simulink model "gm_Model"  (R2025a)
settings: Solver=FixedStepDiscrete  StartTime=0.0  StopTime=80000/fs_in  RelTol=1e-3
undefined symbols (not defined in the file or in its folder): a, b, b_fixp, beta_retanh, c, cos_omega, cos_omega_fixp, diag_count, exp_omega, exp_omega_fixp, fixp_chebacc_frac, fixp_chebacc_ws, fixp_dsp_ws, fixp_eig_frac, fixp_eig_ws, fs_in, group_size, hann_table_fixp, image_seed, image_seed_fixp, J_ROM, k, K_ROM, lap_diags, lap_main, lap_main_fi, lap_offsets, lap_offsets_fi, lap_rest, lap_rest_fi, laplacian_diags_main, laplacian_diags_offsets, laplacian_diags_rest, lut_norm_x, lut_norm_y, magnitude, n_ch, n_layer, n_px, n_px_fi, nf, norm_gain_floor, power_iters, power_norm_scaling_factor_fixp, tau, tau_fixp, theta, theta_fixp
libraries: simulink x59, hdlsllib x36, hdlstreaminglib x4, hdlmdlgenlib x1, matrix_library x1, dspvision x1
(part 8 of 8)

== system gm_Model/DUT_Test/Goertzel/EnabledGoertzel/streaming_partition_streamed2/tappedDelay ==
  in0 : Inport  OutDataTypeStr=fixdt(1, 18, 13)  SampleTime=3.125e-07
      settings: SignalType=complex
  globalSchedule : EnablePort  OutDataTypeStr=boolean
  StateControl : StateControl  StateControl=Synchronous
  tapped_delay : simulink/Discrete/Tapped Delay  vinit=0  samptime=-1  NumDelays=double(47)  DelayOrder=Oldest  includeCurrent=off
  out0 : Outport  OutDataTypeStr=fixdt(1, 18, 13)  PortDimensions=[47]  SampleTime=3.125e-07  InitialOutput=0
      settings: SignalType=complex
  wires:
  in0/1 -> tapped_delay/1
  tapped_delay/1 -> out0/1

== system gm_Model/DUT_Test/Goertzel/EnabledGoertzel/streaming_partition_streamed2/tappedDelay1 ==
  in0 : Inport  OutDataTypeStr=fixdt(1, 18, 13)  SampleTime=3.125e-07
      settings: SignalType=complex
  globalSchedule : EnablePort  OutDataTypeStr=boolean
  StateControl : StateControl  StateControl=Synchronous
  tapped_delay : simulink/Discrete/Tapped Delay  vinit=0  samptime=-1  NumDelays=double(47)  DelayOrder=Oldest  includeCurrent=off
  out0 : Outport  OutDataTypeStr=fixdt(1, 18, 13)  PortDimensions=[47]  SampleTime=3.125e-07  InitialOutput=0
      settings: SignalType=complex
  wires:
  in0/1 -> tapped_delay/1
  tapped_delay/1 -> out0/1

== system gm_Model/DUT_ref/CrossCor/Grouping/DataValidDownsampler/RisingEdgeDetector ==
  In1 : Inport
  AND : Logic  IconShape=distinctive  AllPortsSameDT=off  OutDataTypeStr=boolean
  Delay1 : Delay  DelayLength=1
  NOT : Logic  Operator=NOT  IconShape=distinctive  AllPortsSameDT=off  OutDataTypeStr=boolean
  Out1 : Outport
  wires:
  Delay1/1 -> NOT/1
  AND/1 -> Out1/1
  NOT/1 -> AND/1
  In1/1 -> AND/2, Delay1/1

== system gm_Model/DUT_ref/Deblurring/Chebyshev/LaplacianMultiply/For Each Subsystem ==
  note: This is too slow in simulation... Might be more suitable for HDL coder though (not checked)
  note: Main Diagonal
  note: Lower triangle
  note: Upper triangle
  ToIterate : Inport  Partition=on  PartitionDimension=1  PartitionWidth=1  PartitionOffset=0
  Image : Inport  Port=2
  Diag : Inport  Port=3
  Offset : Inport  Port=4
  Dot Product : DotProduct  OutDataTypeStr=Inherit: Inherit via internal rule
  Dot Product1 : DotProduct  OutDataTypeStr=Inherit: Inherit via internal rule
  For Each : ForEach  DisableCoverage=on  ShowIterationIndex=on
  IndexedSelector : Subsystem  Commented=on  TreatAsAtomicUnit=on
  MATLAB Function : MATLAB Function  TreatAsAtomicUnit=on
  Product : Product
  Selector{,1,3,5} (4 alike) : Selector  IndexMode=Zero-based  InputPortWidth=n_px  IndexOptions=Index vector (port)  Indices=[1 3]  OutputSizes=1
  Selector4 : Selector  NumberOfDimensions=2  IndexMode=Zero-based  InputPortWidth=n_px  IndexOptions=Select all,Index vector (port)  Indices=[1 3],1  OutputSizes=1,1
  SplitDiagonals : Subsystem
  Sum1 : Sum  Inputs=++|
  Sum2 : Sum  Inputs=-+|  OutDataTypeStr=uint16  SaturateOnIntegerOverflow=on
  Sum3 : Sum  Inputs=+++
  Terminator : Terminator
  Wrap To Zero : hdlsllib/Discontinuities/Wrap To Zero  Threshold=n_px-1
  Image_out : Outport  ConcatenationDimension=1
  wires:
  MATLAB Function/1(out) -> Dot Product/2
  Sum3/1 -> Image_out/1
  Dot Product/1 -> Sum3/3
  Product/1 -> Sum3/1
  Sum2/1 -> Selector5/2
  For Each/1 -> Sum1/2, Selector4/2, Selector1/2, Selector/2, Sum2/2
  Selector5/1 -> Dot Product1/1
  Dot Product1/1 -> Sum3/2
  SplitDiagonals/2(Rest) -> IndexedSelector/1(diags), MATLAB Function/1(data_matrix), Selector4/1
  Offset/1 -> Sum2/1, Sum1/1
  Selector4/1 -> Dot Product1/2
  Selector3/1 -> Dot Product/1
  Wrap To Zero/1 -> IndexedSelector/2(indices), MATLAB Function/2(col_indices), Selector3/2
  Sum1/1 -> Wrap To Zero/1
  ToIterate/1 -> Terminator/1
  SplitDiagonals/1(Main) -> Selector/1
  Selector/1 -> Product/2
  Selector1/1 -> Product/1
  Diag/1 -> SplitDiagonals/1(Diag)
  Image/1 -> Selector5/1, Selector3/1, Selector1/1

== system gm_Model/DUT_ref/Goertzel/EnabledGoertzel/Goertzel filter/For All Bins Filter ==
  In1 : Inport
  Delay : Delay  DelayLength=1
  Delay1 : Delay  DelayLength=1
  For Each : ForEach  DisableCoverage=on  IterateSubsysMaskParameter=on,on  SubsysMaskParameterIterationDimension=2,2
  Multiply1 : Gain  Gain=cos_omega
  Multiply2 : Gain  Gain=exp_omega
  Sum : Sum  Inputs=++-
  Sum1 : Sum  Inputs=|-+
  Out1 : Outport  ConcatenationDimension=1
  wires:
  Delay/1 -> Sum1/2, Sum/3
  Delay1/1 -> Multiply1/1, Multiply2/1, Delay/1
  Multiply2/1 -> Sum1/1
  Multiply1/1 -> Sum/1
  Sum1/1 -> Out1/1
  Sum/1 -> Delay1/1
  In1/1 -> Sum/2

== system gm_Model/DUT_ref/Deblurring/Chebyshev/LaplacianMultiply/For Each Subsystem/IndexedSelector ==
  diags : Inport  Partition=on  PartitionDimension=1  PartitionWidth=1  PartitionOffset=0
  indices : Inport  Port=2  Partition=on  PartitionDimension=1  PartitionWidth=1  PartitionOffset=0
  For Each : ForEach  DisableCoverage=on
  Selector : Selector  IndexMode=Zero-based  InputPortWidth=n_px  IndexOptions=Index vector (port)  Indices=[1 3]  OutputSizes=1
  selected : Outport  ConcatenationDimension=1
  wires:
  diags/1 -> Selector/1
  Selector/1 -> selected/1
  indices/1 -> Selector/2

== system gm_Model/DUT_ref/Deblurring/Chebyshev/LaplacianMultiply/For Each Subsystem/SplitDiagonals ==
  Diag : Inport
  Selector1 : Selector  NumberOfDimensions=2  InputPortWidth=n_laplacian_diags  IndexOptions=Index vector (dialog),Select all  Indices=1,1  OutputSizes=1,1
  Selector2 : Selector  NumberOfDimensions=2  InputPortWidth=n_laplacian_diags  IndexOptions=Index vector (dialog),Select all  Indices=2:diag_count+1,1  OutputSizes=1,1
  Main : Outport
  Rest : Outport  Port=2
  wires:
  Selector2/1 -> Rest/1
  Selector1/1 -> Main/1
  Diag/1 -> Selector1/1, Selector2/1

== matlab function gm_Model/Unused blocks/LapMultiply ==
  settings: fimath=hdlfimath;
  data: image_in input; out output; lap_main parameter; lap_offsets_fi parameter; n_px_fi parameter; lap_rest parameter
function out = lap_mult(image_in, lap_main, lap_offsets_fi, n_px_fi, lap_rest)
%#codegen
% Assumes col_indices is zero-based, valid, and fixed-size.

out = zeros(size(image_in,1),1,'like', image_in);

for index = 0:n_px_fi-1

    % Main Diagonal
    main1 = image_in(index+1);
    main2 = lap_main;
    
    main = main1 * main2;
    
    % Lower triangle
    index_sat = fi(index, 'OverflowAction','Saturate');
    lap_offsets_sat = fi(lap_offsets_fi, 'OverflowAction','Saturate');
    image_indices = index_sat - lap_offsets_sat;

    low1 = image_in(image_indices+1);
    low2 = lap_rest(:,index+1);
    
    lower = sum(low1.*low2);
     
    % Upper triangle
    MAX_ROWS = size(lap_rest, 1);
    up1 = zeros(MAX_ROWS, 1);
    
    indices_image = index + lap_offsets_fi;
    
    % Set non-existing indices to zero
    coder.unroll();
    for i = 1:MAX_ROWS
        if indices_image(i) > n_px_fi - 1
            indices_image(i) = 0;
        end
    end
    
    coder.unroll();
    for i = 1:MAX_ROWS
        up1(i) = lap_rest(i, indices_image(i) + 1);  % zero-based to 1-based
    end
    up2 = image_in(indices_image+1);
    
    upper = sum(up1.*up2);
    
    % SUM
    out(index+1) = main + lower + upper;

end

== matlab function gm_Model/DUT_ref/Deblurring/Chebyshev/LaplacianMultiply/For Each Subsystem/MATLAB Function ==
  data: data_matrix input; out output; col_indices input
function out = select_elements(data_matrix, col_indices)
%#codegen
% Assumes col_indices is zero-based, valid, and fixed-size.

MAX_ROWS = size(data_matrix, 1);
out = zeros(MAX_ROWS, 1);

coder.unroll();
for i = 1:MAX_ROWS
    out(i) = data_matrix(i, col_indices(i) + 1);  % zero-based to 1-based
end

== matlab function gm_Model/Unused blocks/BackprojOpt/MATLAB Function ==
  data: A input; y output
function y = diag_vec(A)
%#codegen
y = diag(A);

== matlab function gm_Model/Unused blocks/For Each Subsystem/MainDiagonal ==
  settings: fimath=|
      | fimath(...
      |     'RoundMode', 'floor',...
      |     'OverflowMode', 'Saturate',...
      |     'ProductMode', 'FullPrecision', 'ProductWordLength', 32,...
      |     'SumMode', 'FullPrecision', 'SumWordLength', 32,...
      |     'CastBeforeSum', true);
  data: image_in input; out output; index input; laplacian_diags_main parameter; laplacian_diags_offsets parameter; n_px_fi parameter; laplacian_diags_rest parameter
function out = select_elements(image_in, index, laplacian_diags_main, laplacian_diags_offsets, n_px_fi, laplacian_diags_rest)
%#codegen
% Assumes col_indices is zero-based, valid, and fixed-size.


% Main Diagonal

main1 = image_in(index+1);
main2 = laplacian_diags_main(index+1);

main = main1 * main2;



% Lower triangle

image_indices = index - laplacian_diags_offsets;
low1 = image_in(image_indices+1);

low2 = laplacian_diags_rest(:,index+1);

lower = sum(low1.*low2);



% Upper triangle

MAX_ROWS = size(laplacian_diags_rest, 1);
up1 = zeros(MAX_ROWS, 1);

indices_image = index + laplacian_diags_offsets;

% Set non-existing indices to zero
coder.unroll();
for i = 1:MAX_ROWS
    if indices_image(i) > n_px_fi - 1
        indices_image(i) = 0;
    end
end

coder.unroll();
for i = 1:MAX_ROWS
    up1(i) = laplacian_diags_rest(i, indices_image(i) + 1);  % zero-based to 1-based
end

up2 = image_in(indices_image+1);

upper = sum(up1.*up2);

% SUM

out = main + lower + upper;

== matlab function gm_Model/DUT_FixP/Deblurring/Chebyshev/LaplacianMultiply/LapMultiplyFi ==
  settings: fimath=hdlfimath;
  data: image_in input; out output; lap_main_fi parameter; lap_offsets_fi parameter; n_px_fi parameter; lap_rest_fi parameter
function out = lap_mult(image_in, lap_main_fi, lap_offsets_fi, n_px_fi, lap_rest_fi)
%#codegen
% Assumes col_indices is zero-based, valid, and fixed-size.

T_in = coder.const(numerictype(image_in));
diag_count = coder.const(int32(size(lap_rest_fi, 1)));

out = zeros(size(image_in,1),1,'like', image_in);


for index = 0:n_px_fi-1

    % Main Diagonal
    main1 = image_in(index+1);
    main2 = lap_main_fi;
    
    main = fi(main1 * main2, T_in);
    
    % Lower triangle
    index_sat = fi(index, 'OverflowAction','Saturate');
    lap_offsets_sat = fi(lap_offsets_fi, 'OverflowAction','Saturate');
    image_indices = index_sat - lap_offsets_sat;

    low1 = image_in(image_indices+1);
    low2 = lap_rest_fi(:,index+1);
    
    lower = fi(sum(low1.*low2), T_in);
     
    % Upper triangle
    up1 = zeros(diag_count, 1, 'like', lap_rest_fi);
    
    indices_image = index + lap_offsets_fi;
    
    % Set non-existing indices to zero
    coder.unroll();
    for i = 1:diag_count
        if indices_image(i) > n_px_fi - 1
            indices_image(i) = 0;
        end
    end
    
    coder.unroll();
    for i = 1:diag_count
        up1(i) = lap_rest_fi(i, indices_image(i) + 1);  % zero-based to 1-based
    end
    up2 = image_in(indices_image+1);
    
    upper = fi(sum(up1.*up2), T_in);
    
    % SUM
    out(index+1) = main - lower - upper;

end

== matlab function gm_Model/DUT_FixP/CrossCor/NormalizationPower/Diag ==
  data: u input; y output
function y = fcn(u)
%#codegen

y = diag(u);
